simulink model "model_plane_identification_script_v1"  (R2015b)
settings: Solver=FixedStepDiscrete  StartTime=0.0  StopTime=20  RelTol=1e-3
values from neighbouring files (symbols this model uses):
  Aa = Amp_list(ii)    [amplitude_influence.m]    (also in datas.m = 1; model_validation.m = Amp_aileron2)
  Ae = Amp_list(ii)    [amplitude_influence.m]    (also in datas.m = 1; model_validation.m = Amp_elevator2)
  Ar = Amp_list(ii)    [amplitude_influence.m]    (also in datas.m = 1; model_validation.m = Amp_rudder2)
  b = 59.74    [datas.m]
  cbar = 8.32    [datas.m]
  K_wind = [0 0 0 0 0 0]'    [datas.m]
  m = 288772    [datas.m]
  Offset_Accelerometer = 57*10^-6    (= 5.7e-05)    [datas.m]
  Offset_gyro = 0.15/180*pi    (= 0.00261799387799)    [datas.m]
  Offset_velocity_angles = 0.1/180*pi    (= 0.00174532925199)    [datas.m]
  S = 510.95    [datas.m]
  Ta = 6    [datas.m]
  Te = 4    [datas.m]
  test_aileron = 1    [datas.m]    (also in model_validation.m = aileron2)
  test_elevator = 4    [datas.m]    (also in model_validation.m = elevator2)
  test_rudder = 1    [datas.m]    (also in model_validation.m = rudder2)
  Tr = 2    [datas.m]
undefined symbols (not defined in the file or in its folder): airlib, B747, DiscIntNeverNeededParam, DT, sigbuilder_block
undefined symbols (not defined in the file): Cd_0_true, Cd_alpha_true, Cd_deltae_true, Cd_q_true, Cdih_true, Cl_0_true, CL_0_true, CL_alpha_true, Cl_b_true, Cl_deltaa_true, CL_deltae_true, Cl_deltar_true, Cl_p_true, CL_q_true, Cl_r_true, CLih_true, Cm_0_true, Cm_alpha_true, Cm_deltae_true, Cm_ih_true, Cm_q_true, Cn_0_true, Cn_b_true, Cn_deltaa_true, Cn_deltar_true, Cn_p_true, Cn_r_true, Cy_0_true, Cy_b_true, Cy_deltaa_true, Cy_deltar_true, Cy_p_true, Cy_r_true, Ix, Iy, Iz, Jxy, Jxz, Jyz, V
libraries: simulink x4
(part 1 of 2)
settings Model: Creator=LiMing  LastModifiedBy=c.mathis
settings DataIOCC: LimitDataPoints=off  SaveFormat=Array  SignalLoggingSaveFormat=ModelDataLogs  SaveOutput=off  SaveTime=off
settings OptimizationCC: BlockReduction=off  BooleanDataType=off  ExpressionDepthLimit=2147483647  InitFltsAndDblsToZero=on
settings DebuggingCC: SaveWithParameterizedLinksMsg=none  UnderspecifiedInitializationDetection=Classic  MergeDetectMultiDrivingBlocksExec=none  SignalResolutionControl=TryResolveAllWithWarning  MultiTaskDSMMsg=warning  MultiTaskCondExecSysMsg=none  FcnCallInpInsideContextMsg=UseLocalSettings  StateNameClashWarn=warning
settings HardwareCC: ProdBitPerPointer=32  ProdLargestAtomicFloat=None  ProdIntDivRoundTo=Undefined  ProdEndianess=Unspecified  ProdWordSize=32  ProdHWDeviceType=32-bit Generic  TargetUnknown=on
settings GRTTargetCC: GeneratePreprocessorConditionals=Disable all  CombineOutputUpdateFcns=off  GRTInterface=on
settings ConfigComp: CovModelRefEnable=Off

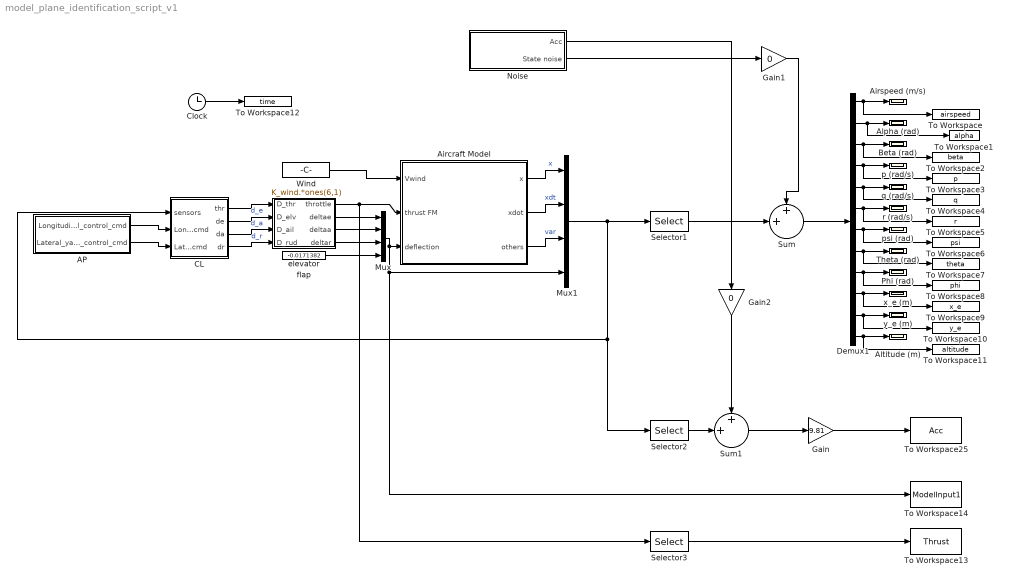
== system model_plane_identification_script_v1 ==
  AP : Subsystem
  Aircraft Model : Subsystem  AncestorBlock=airlib/DT-B747  mask(Discrete Time General Nonlinear Aircraft Model){GM1=[cbar   b   S   Ix  Iy   Iz   Jxy   Jxz  Jyz   m  0.02], CD_wind=[Cd_0_true  Cd_alpha_true  Cd_q_true  Cd_deltae_true  Cdih_true], CL_wind=[CL_0_true  CL_alpha_true  CL_q_true  CL_deltae_true  CLih_true], Cm_body=[Cm_0_true  Cm_alpha_true   Cm_q_true  Cm_deltae_true  Cm_ih_true ], CY_body=[Cy_0_true   Cy_b_true    Cy_p_true     Cy_r_true     Cy_deltaa_true    Cy_deltar_true], Cl_body=[Cl_0_true    Cl_b_true    Cl_p_true   Cl_r_true   Cl_deltaa_true   Cl_deltar_true], Cn_body=[Cn_0_true    Cn_b_true   Cn_p_true    Cn_r_true     Cn_deltaa_true   Cn_deltar_true], x0=[V  0.0464959 0   0 0 0   0 0.0464959 0   0 0 61]}
      mask prompts: GM1 "Geometry, Mass, T : [cbar   b    S    Ix   Iy   Iz   Jxy  Jxz  Jyz  m  T]"; CD_wind "Aerodynamic D-Force Derivatives : [CD0 CDa CDq CDde CDih]"; CL_wind "Aerodynamic L-Force Derivatives : [CL0 CLa CLq CLde CLih]"; Cm_body "Aerodynamic Y-Moment Derivatives : [Cm0 Cma Cmq Cmde Cmih]"; CY_body "Aerodynamic Y-Force Derivatives : [CY0 CYb CYp CYr CYda CYdr]"; Cl_body "Aerodynamic X-moment Derivatives : [Cl0 Clb Clp Clr Clda Cldr]"; Cn_body "Aerodynamic Z-moment Derivatives : [Cn0 Cnb Cnp Cnr Cnda Cndr]"; x0 "Initial Condition x0 [v alpha beta p q r psi theta phi xe ye H]"
      mask help:
      | The first input contains the wind velocity and acceleration.
      |   The second input contains external forces and moments in body axis.
      |   The third input contains the deflections of elevators, ailerons, rudder,
      |   and flaps. For a list of outputs look under the mask.
      |   NB : The International measurement system (MKS) is adopted.
      mask init:
      | AM=zeros(6,19);
      | AM(1,[1 2 9 11 12])=reshape(CD_wind,1,5);
      | AM(3,[1 2 9 11 12])=reshape(CL_wind,1,5);
      | AM(5,[1 2 9 11 12])=reshape(Cm_body,1,5);
      | AM(2,[1 5 8 10 13 14])=reshape(CY_body,1,6);
      | AM(4,[1 5 8 10 13 14])=reshape(Cl_body,1,6);
      | AM(6,[1 5 8 10 13 14])=reshape(Cn_body,1,6);
      | 
      | Ix=GM1(4);Iy=GM1(5);Iz=GM1(6);
      | Jxy=GM1(7);Jxz=GM1(8);Jyz=GM1(9);
      | 
      | detI = Ix*Iy*Iz - 2*Jxy*Jxz*Jyz - Ix*Jyz^2 - Iy*Jxz^2 - Iz*Jxy^2;
      | I1   = Iy*Iz - Jyz^2;I2   = Jxy*Iz + Jyz*Jxz;
      | I3   = Jxy*Jyz + Iy*Jxz;I4   = Ix*Iz - Jxz^2;
      | I5   = Ix*Jyz + Jxy*Jxz;I6   = Ix*Iy - Jxy^2;
      | 
      | Pl  = I1/detI; Pm = I2/detI; Pn = I3/detI;
      | Ppp = -(Jxz*I2 - Jxy*I3)/detI;Ppq = (Jxz*I1 - Jyz*I2 - (Iy-Ix)*I3)/detI;
      | Ppr = -(Jxy*I1 + (Ix-Iz)*I2 - Jyz*I3)/detI;Pqq = (Jyz*I1 - Jxy*I3)/detI;
      | Pqr = -((Iz-Iy)*I1 - Jxy*I2 + Jxz*I3)/detI;Prr = -(Jyz*I1 - Jxz*I2)/detI;
      | 
      | Ql  = I2/detI; Qm = I4/detI; Qn = I5/detI;
      | Qpp = -(Jxz*I4 - Jxy*I5)/detI;Qpq = (Jxz*I2 - Jyz*I4 - (Iy-Ix)*I5)/detI;
      | Qpr = -(Jxy*I2 + (Ix-Iz)*I4 - Jyz*I5)/detI;Qqq = (Jyz*I2 - Jxy*I5)/detI;
      | Qqr = -((Iz-Iy)*I2 - Jxy*I4 + Jxz*I5)/detI;Qrr = -(Jyz*I2 - Jxz*I4)/detI;
      | 
      | Rl  = I3/detI; Rm = I5/detI; Rn = I6/detI;
      | Rpp = -(Jxz*I5 - Jxy*I6)/detI;
      | Rpq = (Jxz*I3 - Jyz*I5 - (Iy-Ix)*I6)/detI;
      | Rpr = -(Jxy*I3 + (Ix-Iz)*I5 - Jyz*I6)/detI;
      | Rqq = (Jyz*I3 - Jxy*I6)/detI;
      | Rqr = -((Iz-Iy)*I3 - Jxy*I5 + Jxz*I6)/detI;
      | Rrr = -(Jyz*I3 - Jxz*I5)/detI;
      | 
      | GM2 = [  Pl   Pm   Pn   Ppp  Ppq  Ppr  Pqq  Pqr  Prr ;
      |                Ql  Qm   Qn   Qpp  Qpq  Qpr  Qqq  Qqr  Qrr ;
      |                Rl  Rm   Rn   Rpp  Rpq  Rpr  Rqq  Rqr  Rrr ];
      | 
      | xfix=1;
      | T=GM1(11);
      mask Help:
      | <p>
      | This block is a general nonlinear 6DOF aircraft model, with a very accurate built-in atmosphere model and constant aerodynamic derivatives.
      | The architecture of the block is largely based on the Aircraft block provided by the <A
      | HREF="http://www.mathworks.com/matlabcentral/fileexchange/loadFile.do?objectId=252&objectType=file">FDC toolbox</A> (Marc Rauw, 1993-2000).
      | </p>
      | <p>
      | The geometric and inertal data of the aircraft are entered as parameters in the first row of the mask, sampling time is the last parameter. The other six rows contains the non-dimensional aerodynamic derivatives. The last row is the initial state.
      | </p>
      | <p>
      | The first input contains the wind velocity and acceleration.
      | The second input contains external forces and moments in the aircraft body axis.
      | The third input contains the deflections of elevators, ailerons, rudder,
      | and flaps or stabilators. For a list of outputs look under the mask.
      | </p>
      | <p>
      | The control surface sign conventions are the same adopted in books such as Stevens-Lewis and Etkin, and in many flight simulators,
      | including the FDC toolbox. <br>
      | Specifically, positive elevator deflection causes negative pitching moment (Cmde &#60 0), positive rudder deflection causes negative yawing
      | moment (Cndr &#60 0), and positive aileron deflection causes negative rolling moment (Clda &#60 0). Another way to say the same thing is
      | that, the positive elevators deflection is Trailing Edge Down (TED), the positive rudder(s) deflection is Trailing Edge Left (TEL), and,
      | taking as TED the positive ailerons deflection, da=K*(da_right-da_left), with K usually equal to 1 (FDC) or 1/2.
      | </p>
      | <p>
      | Since this block is largely based on the FDC toolbox, i redirect you to the FDC Toolbox manual, for a good explanation of the underlying
      | components. Besides the mask and the fact that the aerodynamic derivatives are expressed in the stability axis, the only relevant difference
      | with the FDC toolbox is that in the computation of the aerodynamic forces, q is normalized as q*cbar/2V instead of q*cbar/V. The majority
      | of aeronautics books that i've seen use q*cbar/2V.
      | </p>
      | <p>
      | Please note that the International Measurement System is adopted. So, lengths are in meters, masses in Kg, and inertia moments in Kg*m^2.
      | Moreover, forces are in N, moments in N*m, accelerations in g, and angles in radians. For those that use the english system, here are some useful
      | conversion factors: <br>
      | 1 ft   = 0.3048 m, 1 lb   = 0.4536 Kg, 1 slug = 14.593903 Kg ,  1 slug*ft^2 = 1.355818 Kg*m^2
      | <br>
      | </p>
      | <p>
      | Finally, there is an <A HREF="http://www.aae.uiuc.edu/m-selig/apasim/Aircraft-uiuc.html">excellent source</A> of aircraft aerodynamic data
      | which is mantained by Michael S. Selig, Rob Deters, and Glen Dimock at the university of Urbana-Champaign. To use any of the given models
      | you just need to type the supplied aircraft data in the block mask.
      | </p>
      | <p>
      | <p>
      | December 2002, Giampiero Campa
      | </p>
      | </p>
      mask Display:
      | image(imread('ATR72.jpg'))
      | %disp('Discrete\nTime\nGeneral\nAircraft\nModel')
  Airspeed (m/s) : Scope
  Alpha (rad) : Scope
  Altitude (m) : Scope
  Beta (rad) : Scope
  CL : Subsystem
  Clock : Clock
      settings: Decimation=20
  Demux1 : Demux  Outputs=12
  Gain : Gain  Gain=9.81
  Gain1 : Gain  Gain=0
  Gain2 : Gain  Gain=0
  Mux : Mux
  Mux1 : Mux  Inputs=[12 12 9 4]
  Noise : Subsystem
  Phi (rad) : Scope
  Selector1 : Selector  InputPortWidth=37  IndexOptions=Index vector (dialog)  Indices=1:12  OutputSizes=1
  Selector2 : Selector  InputPortWidth=37  IndexOptions=Index vector (dialog)  Indices=28:30  OutputSizes=1
  Selector3 : Selector  InputPortWidth=6  IndexOptions=Index vector (dialog)  Indices=1  OutputSizes=1
  Sum : Sum  Inputs=++|
  Sum1 : Sum  Inputs=++|
  Theta (rad) : Scope
  To Workspace : ToWorkspace  VariableName=airspeed  SampleTime=-1
  To Workspace1 : ToWorkspace  VariableName=alpha  SampleTime=-1
  To Workspace10 : ToWorkspace  VariableName=y_e  SampleTime=-1
  To Workspace11 : ToWorkspace  VariableName=altitude  SampleTime=-1
  To Workspace12 : ToWorkspace  VariableName=time  SampleTime=-1
  To Workspace13 : ToWorkspace  VariableName=Thrust  SaveFormat=Structure With Time  SampleTime=-1
  To Workspace14 : ToWorkspace  VariableName=ModelInput1  SaveFormat=Structure With Time  SampleTime=-1
  To Workspace2 : ToWorkspace  VariableName=beta  SampleTime=-1
  To Workspace25 : ToWorkspace  VariableName=Acc  SampleTime=-1
  To Workspace3 : ToWorkspace  VariableName=p  SampleTime=-1
  To Workspace4 : ToWorkspace  VariableName=q  SampleTime=-1
  To Workspace5 : ToWorkspace  VariableName=r  SampleTime=-1
  To Workspace6 : ToWorkspace  VariableName=psi  SampleTime=-1
  To Workspace7 : ToWorkspace  VariableName=theta  SampleTime=-1
  To Workspace8 : ToWorkspace  VariableName=phi  SampleTime=-1
  To Workspace9 : ToWorkspace  VariableName=x_e  SampleTime=-1
  Wind : Constant  Value=K_wind.*ones(6,1)
  elevator : Subsystem
      mask Display: disp('Engine &\nCable &\nActuator')
  flap : Constant  Value=-0.0171382
  p (rad/s) : Scope
  psi (rad) : Scope
  q (rad/s) : Scope
  r (rad/s) : Scope
  x_e (m) : Scope
  y_e (m) : Scope
  wires:
  elevator/3(deltaa) -> Mux/2
  elevator/4(deltar) -> Mux/3
  elevator/2(deltae) -> Mux/1
  CL/2(de) -> elevator/2(D_elv)  "d_e"
  CL/3(da) -> elevator/3(D_ail)  "d_a"
  CL/4(dr) -> elevator/4(D_rud)  "d_r"
  elevator/1(throttle) -> Aircraft Model/2(thrust FM), Selector3/1
  Demux1/1 -> Airspeed (m/s)/1, To Workspace/1
  Demux1/2 -> To Workspace1/1, Alpha (rad)/1
  Demux1/3 -> Beta (rad)/1, To Workspace2/1
  Demux1/5 -> q (rad/s)/1, To Workspace4/1
  Demux1/6 -> r (rad/s)/1, To Workspace5/1
  Demux1/7 -> psi (rad)/1, To Workspace6/1
  Demux1/8 -> Theta (rad)/1, To Workspace7/1
  Demux1/9 -> Phi (rad)/1, To Workspace8/1
  Demux1/10 -> x_e (m)/1, To Workspace9/1
  Demux1/11 -> y_e (m)/1, To Workspace10/1
  Demux1/12 -> Altitude (m)/1, To Workspace11/1
  CL/1(thr) -> elevator/1(D_thr)
  flap/1 -> Mux/4
  Wind/1 -> Aircraft Model/1(" Vwind")
  Aircraft Model/1(x) -> Mux1/1  "x"
  Aircraft Model/2(xdot) -> Mux1/2  "xdt"
  Aircraft Model/3(others) -> Mux1/3  "var"
  Clock/1 -> To Workspace12/1
  AP/1(Longitudinal_control_cmd) -> CL/2(Longitudinal_control_cmd)
  AP/2(Lateral_yaw_control_cmd) -> CL/3(Lateral_yaw_control_cmd)
  Selector2/1 -> Sum1/2
  Gain/1 -> To Workspace25/1
  Mux1/1 -> CL/1(sensors), Selector2/1, Selector1/1
  Sum/1 -> Demux1/1
  Selector1/1 -> Sum/2
  Sum1/1 -> Gain/1
  Mux/1 -> To Workspace14/1, Mux1/4, Aircraft Model/3(deflection)
  Selector3/1 -> To Workspace13/1
  Noise/1("Acc ") -> Gain2/1
  Demux1/4 -> p (rad/s)/1, To Workspace3/1
  Noise/2(State noise) -> Gain1/1
  Gain2/1 -> Sum1/1
  Gain1/1 -> Sum/1

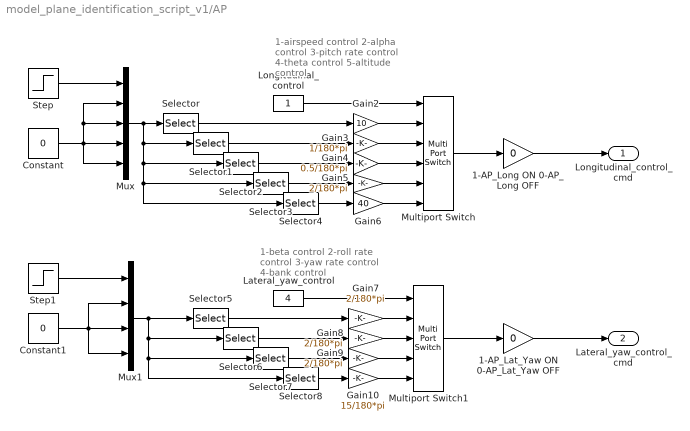
== system model_plane_identification_script_v1/AP ==
  note: 1-airspeed control
      | 2-alpha control
      | 3-pitch rate control
      | 4-theta control
      | 5-altitude control
  note: 1-beta control
      | 2-roll rate control
      | 3-yaw rate control
      | 4-bank control
  1-AP_Lat_Yaw ON 0-AP_Lat_Yaw OFF : Gain  Gain=0
  1-AP_Long ON 0-AP_Long OFF : Gain  Gain=0
  Constant : Constant  Value=0
  Constant1 : Constant  Value=0
  Gain10 : Gain  Gain=15/180*pi
  Gain2 : Gain  Gain=10
  Gain3 : Gain  Gain=1/180*pi
  Gain4 : Gain  Gain=0.5/180*pi
  Gain{5,7..9} (4 alike) : Gain  Gain=2/180*pi
  Gain6 : Gain  Gain=40
  Lateral_yaw_control : Constant  Value=4
  Longitudinal_control : Constant
  Multiport Switch : MultiPortSwitch  Inputs=5
  Multiport Switch1 : MultiPortSwitch  Inputs=4
  Mux : Mux  Inputs=5
  Mux1 : Mux
  Selector : Selector  InputPortWidth=5  IndexOptions=Index vector (dialog)  Indices=[1 2 3 4 5]  OutputSizes=1
  Selector1 : Selector  InputPortWidth=5  IndexOptions=Index vector (dialog)  Indices=[2 1 3 4 5]  OutputSizes=1
  Selector2 : Selector  InputPortWidth=5  IndexOptions=Index vector (dialog)  Indices=[3 2 1 4 5]  OutputSizes=1
  Selector3 : Selector  InputPortWidth=5  IndexOptions=Index vector (dialog)  Indices=[4 2 3 1 5]  OutputSizes=1
  Selector4 : Selector  InputPortWidth=5  IndexOptions=Index vector (dialog)  Indices=[5 2 3 4 1]  OutputSizes=1
  Selector5 : Selector  InputPortWidth=4  IndexOptions=Index vector (dialog)  Indices=[1 2 3 4]  OutputSizes=1
  Selector6 : Selector  InputPortWidth=4  IndexOptions=Index vector (dialog)  Indices=[2 1 3 4]  OutputSizes=1
  Selector7 : Selector  InputPortWidth=4  IndexOptions=Index vector (dialog)  Indices=[3 2 1 4]  OutputSizes=1
  Selector8 : Selector  InputPortWidth=4  IndexOptions=Index vector (dialog)  Indices=[4 2 3 1]  OutputSizes=1
  Step : Step  Time=20  SampleTime=0
  Step1 : Step  Time=20  SampleTime=0
  Longitudinal_control_cmd : Outport
  Lateral_yaw_control_cmd : Outport  Port=2
  wires:
  Step/1 -> Mux/1
  Constant/1 -> Mux/4, Mux/5, Mux/2, Mux/3
  Mux/1 -> Selector/1, Selector1/1, Selector2/1, Selector3/1, Selector4/1
  Selector/1 -> Gain2/1
  Longitudinal_control/1 -> Multiport Switch/1
  Selector1/1 -> Gain3/1
  Selector2/1 -> Gain4/1
  Selector3/1 -> Gain5/1
  Selector4/1 -> Gain6/1
  Multiport Switch/1 -> 1-AP_Long ON 0-AP_Long OFF/1
  Constant1/1 -> Mux1/3, Mux1/2, Mux1/4
  Mux1/1 -> Selector7/1, Selector8/1, Selector6/1, Selector5/1
  Selector5/1 -> Gain7/1
  Lateral_yaw_control/1 -> Multiport Switch1/1
  Selector6/1 -> Gain8/1
  Selector7/1 -> Gain9/1
  Selector8/1 -> Gain10/1
  Multiport Switch1/1 -> 1-AP_Lat_Yaw ON 0-AP_Lat_Yaw OFF/1
  Step1/1 -> Mux1/1
  1-AP_Long ON 0-AP_Long OFF/1 -> Longitudinal_control_cmd/1
  1-AP_Lat_Yaw ON 0-AP_Lat_Yaw OFF/1 -> Lateral_yaw_control_cmd/1
  Gain3/1 -> Multiport Switch/3
  Gain4/1 -> Multiport Switch/4
  Gain5/1 -> Multiport Switch/5
  Gain6/1 -> Multiport Switch/6
  Gain7/1 -> Multiport Switch1/2
  Gain8/1 -> Multiport Switch1/3
  Gain9/1 -> Multiport Switch1/4
  Gain10/1 -> Multiport Switch1/5
  Gain2/1 -> Multiport Switch/2

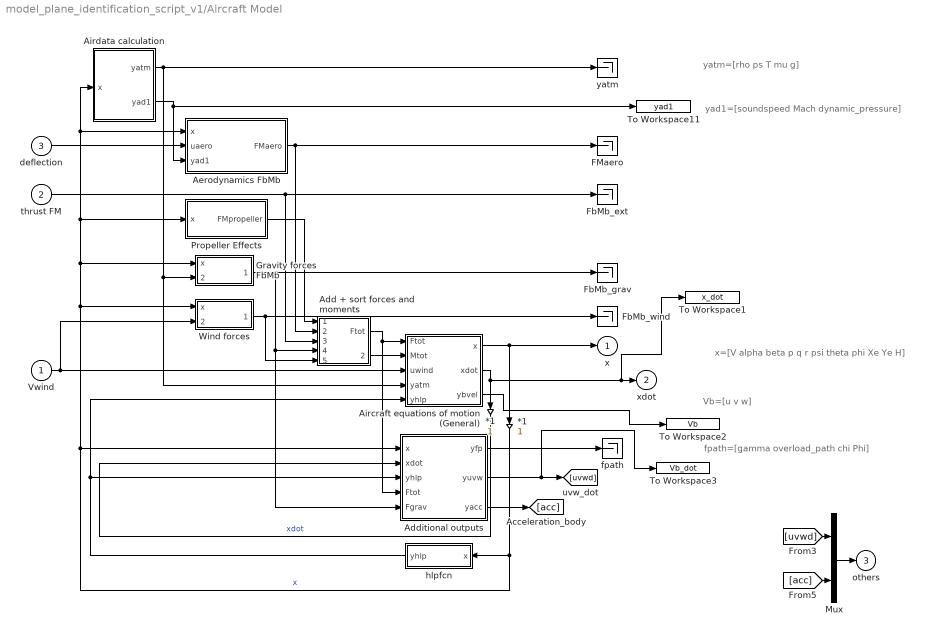
== system model_plane_identification_script_v1/Aircraft Model ==
  note: x=[V alpha beta p q r psi theta phi Xe Ye H]
  note: Vb=[u v w]
  note: fpath=[gamma overload_path chi Phi]
  note: yatm=[rho ps T mu g]
  note: yad1=[soundspeed Mach dynamic_pressure]
  " Vwind" : Inport
  thrust FM : Inport  Port=2
  deflection : Inport  Port=3
  " *1" : Gain  SaturateOnIntegerOverflow=on  OutDataTypeStr=Inherit: Same as input  ParamDataTypeStr=Inherit: Same as input
  *1 : Gain  SaturateOnIntegerOverflow=on  OutDataTypeStr=Inherit: Same as input  ParamDataTypeStr=Inherit: Same as input
  Add + sort forces and moments : Subsystem  mask(FMsort){}
      mask help: Forces and Moments sorting block
      mask Display: disp('FMsort')
  Additional outputs : Subsystem
      mask Display: disp('Additional Outputs')
  Aerodynamics FbMb : Subsystem
      mask Display: disp('Aerodynamics FbMb')
  Aircraft equations of motion (General) : Subsystem
      mask Display: disp('Eqation of Motion')
  Airdata calculation : Subsystem
      mask Display: disp('Airdata')
  FMaero : Terminator
  FbMb_ext : Terminator
  FbMb_grav : Terminator
  FbMb_wind : Terminator
  Gravity forces FbMb : Subsystem  mask(Gravity){m=GM1(10)}
      mask prompts: m "Mass of the aircraft [kg]:"
      mask help: Gravity forces.
      mask Display: disp('Gravity')
  Mux : Mux  Inputs=[3 6]
  Propeller Effects : Subsystem
      mask Display: disp('Propeller Effects')
  To Workspace1 : ToWorkspace  VariableName=x_dot  SampleTime=-1
  To Workspace11 : ToWorkspace  VariableName=yad1  SampleTime=-1
  To Workspace2 : ToWorkspace  VariableName=Vb  SampleTime=-1
  To Workspace3 : ToWorkspace  VariableName=Vb_dot  SampleTime=-1
  Wind forces : Subsystem  mask(fwind){m=GM1(10)}
      mask prompts: m "Mass of the aircraft [kg]:"
      mask help: Forces due to non-steady atmosphere.
      mask Display: disp('Fwind')
  fpath : Terminator
  hlpfcn : Subsystem  mask(Hlpfcn){}
      mask help: Help sines and cosines
      mask Display: disp('hlpfcn')
  yatm : Terminator
  x : Outport
  xdot : Outport  Port=2
  others : Outport  Port=3
  wires:
  Mux/1 -> others/1
  [acc] -> Mux/2
  [uvwd] -> Mux/1
  Additional outputs/2(yuvw) -> To Workspace3/1, [uvwd]
  Add + sort forces and moments/2(Mtot) -> Aircraft equations of motion (General)/2(Mtot)
  Aircraft equations of motion (General)/1(x) -> " *1"/1, x/1
  Aircraft equations of motion (General)/2(xdot) -> *1/1, To Workspace1/1, xdot/1
  " *1"/1 -> Gravity forces FbMb/1(x), Airdata calculation/1(x), Aerodynamics FbMb/1(x), Propeller Effects/1(x), Wind forces/1(x), Additional outputs/1(x), hlpfcn/1(x)  "x"
  Gravity forces FbMb/1(Fgrav) -> FbMb_grav/1, Additional outputs/5(Fgrav), Add + sort forces and moments/4(Fgrav)
  *1/1 -> Additional outputs/2(xdot)  "xdot"
  " Vwind"/1 -> Wind forces/2(uwind), Aircraft equations of motion (General)/3(uwind)
  hlpfcn/1(yhlp) -> Additional outputs/3(yhlp), Aircraft equations of motion (General)/5(yhlp)
  Aerodynamics FbMb/1(FMaero) -> Add + sort forces and moments/2(FMaero), FMaero/1
  Wind forces/1(Fwind) -> Add + sort forces and moments/5(Fwind), FbMb_wind/1
  Additional outputs/3(yacc) -> [acc]
  Airdata calculation/1(yatm) -> yatm/1, Gravity forces FbMb/2(yatm), Aircraft equations of motion (General)/4(yatm)
  Airdata calculation/2(yad1) -> To Workspace11/1, Aerodynamics FbMb/3(yad1)
  Additional outputs/1(yfp) -> fpath/1
  Aircraft equations of motion (General)/3(ybvel) -> To Workspace2/1
  deflection/1 -> Aerodynamics FbMb/2(uaero)
  thrust FM/1 -> FbMb_ext/1, Add + sort forces and moments/3(FMprop)
  Add + sort forces and moments/1(Ftot) -> Aircraft equations of motion (General)/1(Ftot), Additional outputs/4(Ftot)
  Propeller Effects/1(FMpropeller) -> Add + sort forces and moments/1(FM_propeller)

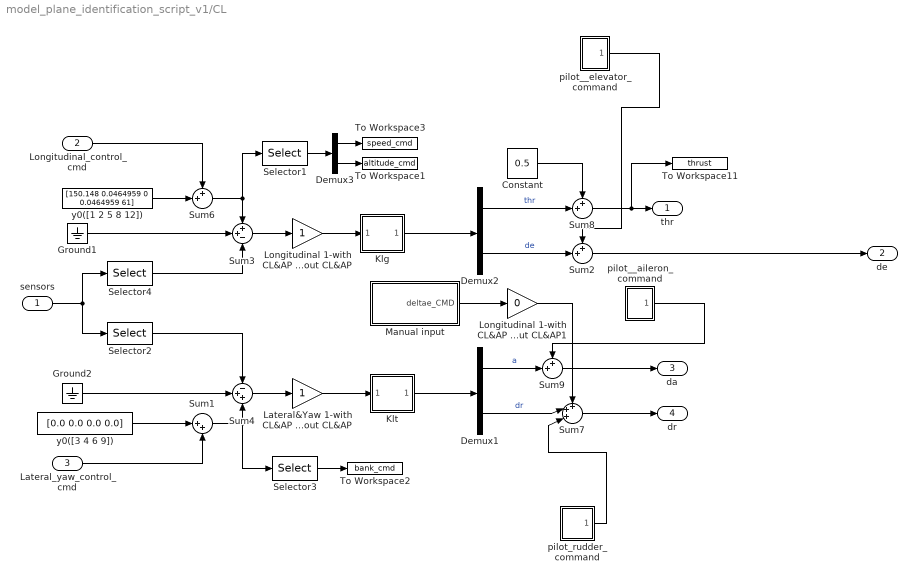
== system model_plane_identification_script_v1/CL ==
  sensors : Inport
  Longitudinal_control_cmd : Inport  Port=2
  Lateral_yaw_control_cmd : Inport  Port=3
  Constant : Constant  Value=0.5
  Demux1 : Demux  Outputs=2
  Demux2 : Demux  Outputs=2
  Demux3 : Demux  Outputs=2
  Ground1 : Ground
  Ground2 : Ground
  "Klg " : Subsystem  mask(State Space){M=[0.1942   -0.8227    0.0057    0.6253    0.0090;  0.0283    7.9374   -5.0871  -16.2986   -0.0437]}
      mask prompts: M "Matrix"
      mask Display: disp('Matrix\nGain')
  "Klt " : Subsystem  mask(State Space){M=[0.2844   -0.1878   -0.2314   -0.1641; 1.1821   -0.4567   -1.8328   -0.4900]}
      mask prompts: M "Matrix"
      mask Display: disp('Matrix\nGain')
  Lateral&Yaw 1-with CL&AP 0-without CL&AP : Gain
  Longitudinal 1-with CL&AP 0-without CL&AP : Gain
  Longitudinal 1-with CL&AP 0-without CL&AP1 : Gain  Gain=0
  Manual input : Subsystem  Tag=STV Subsys  LoadFcn=sigbuilder_block('load');  StartFcn=sigbuilder_block('start');  StopFcn=sigbuilder_block('stop');  ClipboardFcn=sigbuilder_block('clipboard');  mask(Sigbuilder block){}
      mask help: Simulink:masks:SigbuilderBlock_MD
      mask init:
      | if ~strcmp(get_param(bdroot(gcbh),'SimulationStatus'),'stopped') tuvar = sigbuilder_block('maskInit'); end
      settings: CopyFcn=sigbuilder_block('copy');  DeleteFcn=sigbuilder_block('delete');  ModelCloseFcn=sigbuilder_block('modelClose');  PreSaveFcn=sigbuilder_block('preSave');  PauseFcn=sigbuilder_block('pause');  ContinueFcn=sigbuilder_block('continue');  NameChangeFcn=sigbuilder_block('namechange');  OpenFcn=sigbuilder_block('open',[301.5 193.5 843.75 381.75 ]);  CloseFcn=sigbuilder_block('close');
      mask Display: plot(0, 0, 100, 100,[2, 2, 32, 32, 2], [68, 8, 8, 68, 68],[32, 2], [38, 38], [32, 19, 2],[53, 60, 44], [32, 17, 17, 2],[16, 16, 31, 31]);txt = getActiveGroup(gcbh);text(2, 100, txt,'verticalAlignment', 'top');
  Selector1 : Selector  InputPortWidth=5  IndexOptions=Index vector (dialog)  Indices=[1 5]  OutputSizes=1
  Selector2 : Selector  InputPortWidth=37  IndexOptions=Index vector (dialog)  Indices=[3 4 6 9]  OutputSizes=1
  Selector3 : Selector  InputPortWidth=4  IndexOptions=Index vector (dialog)  Indices=[4]  OutputSizes=1
  Selector4 : Selector  InputPortWidth=37  IndexOptions=Index vector (dialog)  Indices=[1 2 5 8 12]  OutputSizes=1
  Sum1 : Sum  Inputs=|++  SaturateOnIntegerOverflow=on  InputSameDT=on  OutDataTypeStr=Inherit: Same as first input
  Sum{2,6,8..9} (4 alike) : Sum  Inputs=++|  SaturateOnIntegerOverflow=on  InputSameDT=on  OutDataTypeStr=Inherit: Same as first input
  Sum3 : Sum  Inputs=++-  SaturateOnIntegerOverflow=on  InputSameDT=on  OutDataTypeStr=Inherit: Same as first input
  Sum4 : Sum  Inputs=-++  SaturateOnIntegerOverflow=on  InputSameDT=on  OutDataTypeStr=Inherit: Same as first input
  Sum7 : Sum  Inputs=+++|  SaturateOnIntegerOverflow=on  InputSameDT=on  OutDataTypeStr=Inherit: Same as first input
  To Workspace1 : ToWorkspace  VariableName=altitude_cmd  SampleTime=-1
  To Workspace11 : ToWorkspace  VariableName=thrust  SampleTime=-1
  To Workspace2 : ToWorkspace  VariableName=bank_cmd  SampleTime=-1
  To Workspace3 : ToWorkspace  VariableName=speed_cmd  SampleTime=-1
  pilot__aileron_command : Subsystem
  pilot__elevator_command : Subsystem
  pilot_rudder_command : Subsystem
  y0([1 2 5 8 12]) : Constant  Value="[150.148  0.0464959 0 0.0464959 61]"
  y0([3 4 6 9]) : Constant  Value=[0.0 0.0 0.0 0.0]
  thr : Outport
  de : Outport  Port=2
  da : Outport  Port=3
  dr : Outport  Port=4
  wires:
  sensors/1 -> Selector4/1, Selector2/1
  Selector4/1 -> Sum3/3
  Sum3/1 -> Longitudinal 1-with CL&AP 0-without CL&AP/1
  Ground1/1 -> Sum3/2
  "Klg "/1(Out1) -> Demux2/1
  Sum4/1 -> Lateral&Yaw 1-with CL&AP 0-without CL&AP/1
  Ground2/1 -> Sum4/2
  Selector2/1 -> Sum4/1
  Lateral_yaw_control_cmd/1 -> Sum1/2
  y0([3 4 6 9])/1 -> Sum1/1
  Sum1/1 -> Sum4/3, Selector3/1
  Longitudinal_control_cmd/1 -> Sum6/1
  y0([1 2 5 8 12])/1 -> Sum6/2
  Sum6/1 -> Sum3/1, Selector1/1
  Longitudinal 1-with CL&AP 0-without CL&AP/1 -> "Klg "/1(In1)
  Manual input/1(deltae_CMD) -> Longitudinal 1-with CL&AP 0-without CL&AP1/1
  Selector1/1 -> Demux3/1
  Demux3/2 -> To Workspace1/1
  Demux3/1 -> To Workspace3/1
  Selector3/1 -> To Workspace2/1
  Demux2/1 -> Sum8/2  "thr"
  Constant/1 -> Sum8/1
  Sum8/1 -> To Workspace11/1, thr/1
  Demux2/2 -> Sum2/2  "de"
  Sum2/1 -> de/1
  pilot__elevator_command/1(Out1) -> Sum2/1
  "Klt "/1(Out1) -> Demux1/1
  Lateral&Yaw 1-with CL&AP 0-without CL&AP/1 -> "Klt "/1(In1)
  Longitudinal 1-with CL&AP 0-without CL&AP1/1 -> Sum7/1
  Demux1/2 -> Sum7/2  "dr"
  Sum7/1 -> dr/1
  pilot_rudder_command/1(Out1) -> Sum7/3
  Demux1/1 -> Sum9/2  "a"
  Sum9/1 -> da/1
  pilot__aileron_command/1(Out1) -> Sum9/1

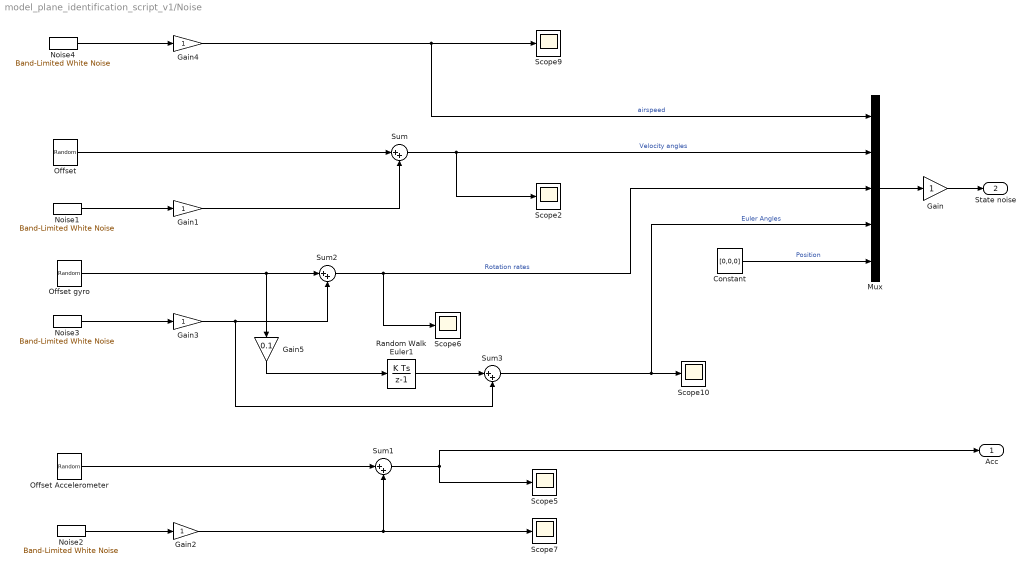
== system model_plane_identification_script_v1/Noise ==
  Constant : Constant  Value=[0,0,0]
  Gain{,1..4} (5 alike) : Gain
  Gain5 : Gain  Gain=0.1
  Mux : Mux  Inputs=5
  Noise1 : simulink/Sources/Band-Limited White Noise  Cov=Noise_power_velocity_angles  Ts=0.02  seed=1:2
  Noise2 : simulink/Sources/Band-Limited White Noise  Cov=Noise_power_Accelerometer  Ts=0.02  seed=2
  Noise3 : simulink/Sources/Band-Limited White Noise  Cov=Noise_power_gyro  Ts=0.02  seed=2
  Noise4 : simulink/Sources/Band-Limited White Noise  Cov=Noise_power_airspeed  Ts=0.02  seed=1
  Offset : UniformRandomNumber  Minimum=-Offset_velocity_angles  Maximum=Offset_velocity_angles  Seed=1:2  SampleTime=0.02
  Offset Accelerometer : UniformRandomNumber  Minimum=-Offset_Accelerometer  Maximum=Offset_Accelerometer  Seed=1:3  SampleTime=0.02
  Offset gyro : UniformRandomNumber  Minimum=-Offset_gyro  Maximum=Offset_gyro  Seed=1:3  SampleTime=0.02
  Random Walk Euler1 : DiscreteIntegrator  gainval=1  InitialConditionSetting=State (most efficient)  SampleTime=-1  ICPrevOutput=DiscIntNeverNeededParam  ICPrevScaledInput=DiscIntNeverNeededParam
  Scope{2,5..7,9..10} (6 alike) : Scope
  Sum{,1..3} (4 alike) : Sum  Inputs=|++
  "Acc " : Outport
  State noise : Outport  Port=2
  wires:
  Noise1/1 -> Gain1/1
  Offset/1 -> Sum/1
  Sum/1 -> Mux/2, Scope2/1  "Velocity angles"
  Noise2/1 -> Gain2/1
  Gain2/1 -> Scope7/1, Sum1/2
  Offset Accelerometer/1 -> Sum1/1
  Noise3/1 -> Gain3/1
  Gain3/1 -> Sum3/2, Sum2/2
  Offset gyro/1 -> Sum2/1, Gain5/1
  Sum2/1 -> Scope6/1, Mux/3  "Rotation rates"
  Sum1/1 -> Scope5/1, "Acc "/1
  Noise4/1 -> Gain4/1
  Gain4/1 -> Mux/1, Scope9/1  "airspeed"
  Constant/1 -> Mux/5  "Position"
  Mux/1 -> Gain/1
  Sum3/1 -> Scope10/1, Mux/4  "Euler Angles"
  Gain1/1 -> Sum/2
  Gain5/1 -> Random Walk Euler1/1
  Random Walk Euler1/1 -> Sum3/1
  Gain/1 -> State noise/1

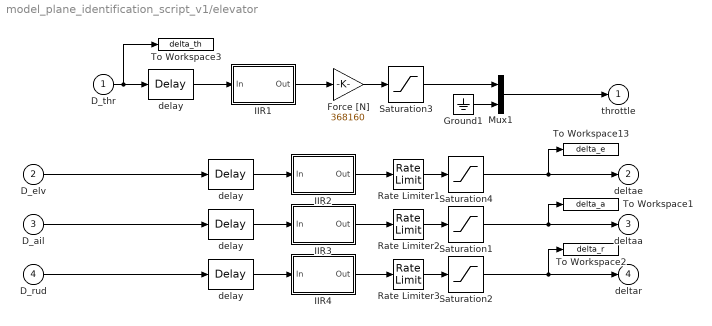
== system model_plane_identification_script_v1/elevator ==
  D_thr : Inport
  D_elv : Inport  Port=2
  D_ail : Inport  Port=3
  D_rud : Inport  Port=4
  " delay" : TransportDelay  DelayTime=0.03  InitialOutput=-1.71374e-004
  " delay " : TransportDelay  DelayTime=0.03  InitialOutput=0.490154
  Force [N] : Gain  Gain=368160  SaturateOnIntegerOverflow=on  OutDataTypeStr=Inherit: Same as input  ParamDataTypeStr=Inherit: Same as input
  Ground1 : Ground
  IIR1 : Subsystem  mask(Discrete Time First Order IIR){ni=1, a=4, x0=0.490154, T=0.02}
      mask prompts: ni "Number of Channels"; a "Cutoff Frequency (a)"; x0 "Initial Condition"; T "Sample Time"
      mask help:
      | Each channel has the transfer function
      |   (1-exp(-aT))/(1-exp(-aT)(z^-1)) which is a good
      |   (pz-matched) approximation of a/(s+a) if 10*a*T<pi
      mask init:
      | A=[];B=[];C=[];D=[];
      | for i=1:ni,
      | A=[A,zeros(size(A,1),1);zeros(1,size(A,2)),exp(-a*T)];
      | B=[B,zeros(size(B,1),1);zeros(1,size(B,2)),1-exp(-a*T)];
      | C=[C,zeros(size(C,1),1);zeros(1,size(C,2)),exp(-a*T)];
      | D=[D,zeros(size(D,1),1);zeros(1,size(D,2)),1-exp(-a*T)];
      | end
      mask Help:
      | <p>
      |   Each channel has the transfer function
      |   (1-exp(-aT))/(1-exp(-aT)(z^-1)) which is a good
      |   (pz-matched) approximation of a/(s+a) if 10*a*T<pi
      | </p>
      mask Display: dpoly(a,[1 a],'s')
  IIR2 : Subsystem  mask(Discrete Time First Order IIR){ni=1, a=15, x0=-1.71374e-004, T=0.02}
      mask prompts: ni "Number of Channels"; a "Cutoff Frequency (a)"; x0 "Initial Condition"; T "Sample Time"
      mask help:
      | Each channel has the transfer function
      |   (1-exp(-aT))/(1-exp(-aT)(z^-1)) which is a good
      |   (pz-matched) approximation of a/(s+a) if 10*a*T<pi
      mask init: same as model_plane_identification_script_v1/elevator/IIR1
      mask Help:
      | <p>
      |   Each channel has the transfer function
      |   (1-exp(-aT))/(1-exp(-aT)(z^-1)) which is a good
      |   (pz-matched) approximation of a/(s+a) if 10*a*T<pi
      | </p>
      mask Display: dpoly(a,[1 a],'s')
  IIR3 : Subsystem  mask(Discrete Time First Order IIR){ni=1, a=15, x0=0, T=0.02}
      mask prompts: ni "Number of Channels"; a "Cutoff Frequency (a)"; x0 "Initial Condition"; T "Sample Time"
      mask help:
      | Each channel has the transfer function
      |   (1-exp(-aT))/(1-exp(-aT)(z^-1)) which is a good
      |   (pz-matched) approximation of a/(s+a) if 10*a*T<pi
      mask init: same as model_plane_identification_script_v1/elevator/IIR1
      mask Help:
      | <p>
      |   Each channel has the transfer function
      |   (1-exp(-aT))/(1-exp(-aT)(z^-1)) which is a good
      |   (pz-matched) approximation of a/(s+a) if 10*a*T<pi
      | </p>
      mask Display: dpoly(a,[1 a],'s')
  IIR4 : Subsystem  mask(Discrete Time First Order IIR){ni=1, a=15, x0=0, T=0.02}
      mask prompts: ni "Number of Channels"; a "Cutoff Frequency (a)"; x0 "Initial Condition"; T "Sample Time"
      mask help:
      | Each channel has the transfer function
      |   (1-exp(-aT))/(1-exp(-aT)(z^-1)) which is a good
      |   (pz-matched) approximation of a/(s+a) if 10*a*T<pi
      mask init: same as model_plane_identification_script_v1/elevator/IIR1
      mask Help:
      | <p>
      |   Each channel has the transfer function
      |   (1-exp(-aT))/(1-exp(-aT)(z^-1)) which is a good
      |   (pz-matched) approximation of a/(s+a) if 10*a*T<pi
      | </p>
      mask Display: dpoly(a,[1 a],'s')
  Mux1 : Mux  Inputs=[1 5]
  Rate Limiter1 : RateLimiter  RisingSlewLimit=100*pi/180  FallingSlewLimit=-100*pi/180
  Rate Limiter2 : RateLimiter  RisingSlewLimit=100*pi/180  FallingSlewLimit=-100*pi/180
  Rate Limiter3 : RateLimiter  RisingSlewLimit=100*pi/180  FallingSlewLimit=-100*pi/180
  Saturation1 : Saturate  UpperLimit=20*pi/180  LowerLimit=-20*pi/180
  Saturation2 : Saturate  UpperLimit=20*pi/180  LowerLimit=-20*pi/180
  Saturation3 : Saturate  UpperLimit=245440  LowerLimit=0
  Saturation4 : Saturate  UpperLimit=20*pi/180  LowerLimit=-20*pi/180
  To Workspace1 : ToWorkspace  VariableName=delta_a  SampleTime=-1
  To Workspace13 : ToWorkspace  VariableName=delta_e  SampleTime=-1
  To Workspace2 : ToWorkspace  VariableName=delta_r  SampleTime=-1
  To Workspace3 : ToWorkspace  VariableName=delta_th  SampleTime=-1
  delay : TransportDelay  DelayTime=0.03
  "delay " : TransportDelay  DelayTime=0.03
  throttle : Outport
  deltae : Outport  Port=2
  deltaa : Outport  Port=3
  deltar : Outport  Port=4
  wires:
  IIR2/1(Out) -> Rate Limiter1/1
  Saturation4/1 -> deltae/1, To Workspace13/1
  IIR3/1(Out) -> Rate Limiter2/1
  Saturation1/1 -> deltaa/1, To Workspace1/1
  IIR4/1(Out) -> Rate Limiter3/1
  Saturation2/1 -> deltar/1, To Workspace2/1
  Rate Limiter1/1 -> Saturation4/1
  Rate Limiter2/1 -> Saturation1/1
  Rate Limiter3/1 -> Saturation2/1
  Saturation3/1 -> Mux1/1
  Ground1/1 -> Mux1/2
  D_thr/1 -> " delay "/1, To Workspace3/1
  IIR1/1(Out) -> Force [N]/1
  Force [N]/1 -> Saturation3/1
  " delay "/1 -> IIR1/1(In)
  " delay"/1 -> IIR2/1(In)
  delay/1 -> IIR3/1(In)
  "delay "/1 -> IIR4/1(In)
  D_elv/1 -> " delay"/1
  D_ail/1 -> delay/1
  D_rud/1 -> "delay "/1
  Mux1/1 -> throttle/1

== system model_plane_identification_script_v1/Aircraft Model/Add + sort forces and moments ==
  FM_propeller : Inport
  FMaero : Inport  Port=2
  FMprop : Inport  Port=3
  Fgrav : Inport  Port=4
  Fwind : Inport  Port=5
  Demux : Demux  Outputs=[3 3]
  Demux1 : Demux  Outputs=[3 3]
  Demux2 : Demux  Outputs=[3 3]
  Sum1 : Sum  Inputs=+++  SaturateOnIntegerOverflow=on  InputSameDT=on  OutDataTypeStr=Inherit: Same as first input
  Sum3 : Sum  Inputs=+++++  SaturateOnIntegerOverflow=on  InputSameDT=on  OutDataTypeStr=Inherit: Same as first input
  Ftot : Outport
  Mtot : Outport  Port=2
  wires:
  Fwind/1 -> Sum3/4
  Demux/1 -> Sum3/1
  Sum1/1 -> Mtot/1
  Sum3/1 -> Ftot/1
  Demux1/1 -> Sum3/2
  Fgrav/1 -> Sum3/3
  Demux/2 -> Sum1/1
  Demux1/2 -> Sum1/2
  FMprop/1 -> Demux1/1
  FMaero/1 -> Demux/1
  FM_propeller/1 -> Demux2/1
  Demux2/1 -> Sum3/5
  Demux2/2 -> Sum1/3

== system model_plane_identification_script_v1/Aircraft Model/Additional outputs ==
  note: Body-axes accelerations
      | and specific forces
  note: du/dt, dv/dt, dw/dt
      | (output equations!)
  note: Flightpath
      | variables
  x : Inport
  xdot : Inport  Port=2
  yhlp : Inport  Port=3
  Ftot : Inport  Port=4
  Fgrav : Inport  Port=5
  accel : Subsystem  mask(accel){m=GM1(10)}
      mask prompts: m "Mass of the aircraft [kg]:"
      mask help:
      | Body axes accelerations and
      | specific forces.
      mask Display: disp('Accel')
  fp : Subsystem  mask(Flpath){alpha0=x0(2)}
      mask prompts: alpha0 "Initial value of angle of attack, alpha0:"
      mask help: Flightpath related parameters.
      mask Display: disp('flpath')
  uvwdot : Subsystem  mask(uvwdot){}
      mask help: Calculation of du/dt, dv/dt, and dw/dt.
      mask Display: disp('uvwdot')
  yfp : Outport
  yuvw : Outport  Port=2
  yacc : Outport  Port=3
  wires:
  Fgrav/1 -> accel/2(Fgrav)
  x/1 -> uvwdot/1(x), fp/1(x)
  xdot/1 -> uvwdot/2(xdot), fp/2(xdot)
  accel/1(yacc) -> yacc/1
  Ftot/1 -> accel/1(Ftot)
  yhlp/1 -> uvwdot/3(yhlp)
  uvwdot/1(yuvw = [udot; vdot; wdot]) -> yuvw/1
  fp/1(yfp) -> yfp/1

== system model_plane_identification_script_v1/Aircraft Model/Aerodynamics FbMb ==
  x : Inport
  uaero : Inport  Port=2
  yad1 : Inport  Port=3
  Caero : Terminator
  aero : Subsystem  mask(Aeromod){}
      mask help: Aerodynamic model of the DHC-2 'Beaver'.
      mask Display: disp('Aeromod\n(General)')
  dl : Subsystem  mask(Dimless){cbar=GM1(1), b=GM1(2)}
      mask prompts: cbar "Mean aerodynamic chord [m]:"; b "Wing span [m]:"
      mask help: Dimensionless rotational velocities.
      mask Display: disp('Dimless')
  fmdims : Subsystem  mask(FMdims){cbar=GM1(1), b=GM1(2), S=GM1(3)}
      mask prompts: cbar "Mean aerodynamic chord [m]:"; b "Wing span [m]:"; S "Wing surface [m^2]:"
      mask help:
      | Calculate forces and moments from
      | dimensionless derivatives.
      mask Display: disp('FMdims')
  ydl : Terminator
  FMaero : Outport
  wires:
  fmdims/1(Forces and moments) -> FMaero/1
  yad1/1 -> fmdims/1(yad1)
  uaero/1 -> aero/2(uaero)
  x/1 -> aero/1(x), dl/1(x)
  dl/1(ydl) -> aero/3(ydl), ydl/1
  aero/1(Caero) -> fmdims/2(Force / moment derivatives), Caero/1

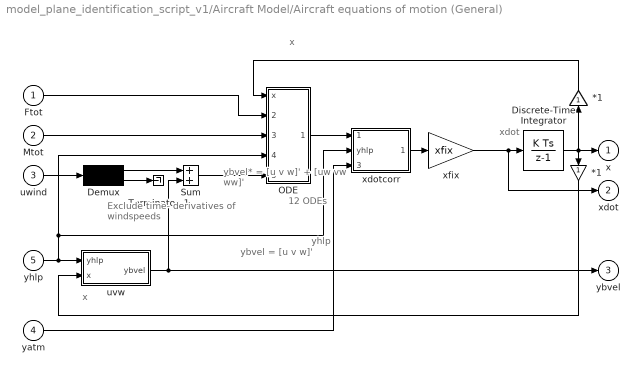
== system model_plane_identification_script_v1/Aircraft Model/Aircraft equations of motion (General) ==
  note: 12 ODEs
  note: ybvel = [u v w]'
  note: yhlp
  note: x
  note: x
  note: xdot
  note: ybvel* =
      | [u v w]' +
      | [uw vw ww]'
  note: Exclude time-
      | derivatives
      | of windspeeds
  Ftot : Inport
  Mtot : Inport  Port=2
  uwind : Inport  Port=3
  yatm : Inport  Port=4
  yhlp : Inport  Port=5
  " *1" : Gain  SaturateOnIntegerOverflow=on  OutDataTypeStr=Inherit: Same as input  ParamDataTypeStr=Inherit: Same as input
  *1 : Gain  SaturateOnIntegerOverflow=on  OutDataTypeStr=Inherit: Same as input  ParamDataTypeStr=Inherit: Same as input
  Demux : Demux  Outputs=[3 3]
  Discrete-Time Integrator : DiscreteIntegrator  InitialCondition=x0  SampleTime=T  ICPrevOutput=DiscIntNeverNeededParam  ICPrevScaledInput=DiscIntNeverNeededParam
  ODE : Subsystem
  Sum : Sum  SaturateOnIntegerOverflow=on  InputSameDT=on  OutDataTypeStr=Inherit: Same as first input
  Terminator_1 : Terminator
  uvw : Subsystem  mask(uvw){}
      mask help:
      | Calculation of body-axes velocities
      | u, v, and w
      mask Display: disp('Body-axes\nvelocities')
  xdotcorr : Subsystem  mask(xdotcorr){b=GM1(2), S=GM1(3), m=GM1(10), CYbdot=AM(2,19)}
      mask prompts: b "Wing span [m]:"; S "Wing surface [m^2]:"; m "Mass of the aircraft [kg]:"; CYbdot "Stability-derivative CYbdot:"
      mask help:
      | Correction block to write state
      | equations for DHC-2 Beaver aircraft
      | explicitly.
      mask Display: disp('xdotcorr\n(General)')
  xfix : Gain  Gain=xfix  SaturateOnIntegerOverflow=on  OutDataTypeStr=Inherit: Same as input  ParamDataTypeStr=Inherit: Same as input
  x : Outport
  xdot : Outport  Port=2
  ybvel : Outport  Port=3
  wires:
  " *1"/1 -> ODE/1(x)
  xfix/1 -> xdot/1, Discrete-Time Integrator/1
  Discrete-Time Integrator/1 -> *1/1, " *1"/1, x/1
  *1/1 -> uvw/2(x)
  Mtot/1 -> ODE/3(Mtot)
  Ftot/1 -> ODE/2(Ftot)
  yatm/1 -> xdotcorr/3(yatm)
  xdotcorr/1(xdot corrected) -> xfix/1
  Demux/1 -> Sum/1
  uwind/1 -> Demux/1
  uvw/1(ybvel) -> Sum/2, ybvel/1
  Sum/1 -> ODE/5(ybvel*)
  ODE/1(xdot) -> xdotcorr/1(xdot uncorrected)
  yhlp/1 -> xdotcorr/2(yhlp), ODE/4(yhlp), uvw/1(yhlp)
  Demux/2 -> Terminator_1/1

== system model_plane_identification_script_v1/Aircraft Model/Airdata calculation ==
  note: yatm=[rho ps T mu g]
  note: yad1=[soundspeed Mach dynamic_pressure]
  x : Inport
  ad1 : Subsystem  mask(Airdata1){}
      mask help: Basic airdata variables
      mask Display: disp('Airdata1')
  ad2 : Subsystem  mask(Airdata2){}
      mask help: More airdata variables
      mask Display: disp('Airdata2')
  ad3 : Subsystem  mask(Airdata3){cbar=GM1(1)}
      mask prompts: cbar "Mean aerodynamic chord [m]:"
      mask help: More airdata variables
      mask Display: disp('Airdata3')
  atm : Subsystem  mask(Atmosph){}
      mask help: Atmosphere variables
      mask Display: disp('Atmosph')
  yad2 : Terminator
  yad3 : Terminator
  yatm : Outport
  yad1 : Outport  Port=2
  wires:
  ad1/1(yad1) -> ad3/3(yad1), ad2/2(yad1), yad1/1
  atm/1(yatm) -> ad3/2(yatm), ad2/1(yatm), ad1/2(yatm), yatm/1
  x/1 -> ad3/1(x), ad1/1(x), atm/1(x)
  ad3/1(yad3) -> yad3/1
  ad2/1(yad2) -> yad2/1

== system model_plane_identification_script_v1/Aircraft Model/Gravity forces FbMb ==
  x : Inport
  yatm : Inport  Port=2
  Mux : Mux  Inputs=3
  Mux1 : Mux  Inputs=[12 5]
  Xgr : Fcn  Expr=-m*u[17]*sin(u[8])
  Ygr : Fcn  Expr=m*u[17]*cos(u[8])*sin(u[9])
  Zgr : Fcn  Expr=m*u[17]*cos(u[8])*cos(u[9])
  Fgrav : Outport
  wires:
  yatm/1 -> Mux1/2
  x/1 -> Mux1/1
  Zgr/1 -> Mux/3
  Mux1/1 -> Zgr/1, Xgr/1, Ygr/1
  Mux/1 -> Fgrav/1
  Ygr/1 -> Mux/2
  Xgr/1 -> Mux/1

== system model_plane_identification_script_v1/Aircraft Model/Propeller Effects ==
  x : Inport
  Constant : Constant  Value=0
  Mux1 : Mux  Inputs=6
  xt : Terminator
  FMpropeller : Outport
  wires:
  Constant/1 -> Mux1/1, Mux1/2, Mux1/3, Mux1/4, Mux1/5, Mux1/6
  Mux1/1 -> FMpropeller/1
  x/1 -> xt/1

== system model_plane_identification_script_v1/Aircraft Model/Wind forces ==
  x : Inport
  uwind : Inport  Port=2
  -Xw/m : Fcn  Expr=u[16] + u[5]*u[15] - u[6]*u[14]
  -Yw/m : Fcn  Expr=u[17] - u[4]*u[15] + u[6]*u[13]
  -Zw/m : Fcn  Expr=u[18] + u[4]*u[14] - u[5]*u[13]
  Mux : Mux  Inputs=3
  Mux1 : Mux  Inputs=[12 6]
  gain : Gain  Gain=-m  SaturateOnIntegerOverflow=on  OutDataTypeStr=Inherit: Same as input  ParamDataTypeStr=Inherit: Same as input
  Fwind : Outport
  wires:
  -Zw/m/1 -> Mux/3
  -Xw/m/1 -> Mux/1
  -Yw/m/1 -> Mux/2
  Mux1/1 -> -Xw/m/1, -Zw/m/1, -Yw/m/1
  Mux/1 -> gain/1
  gain/1 -> Fwind/1
  x/1 -> Mux1/1
  uwind/1 -> Mux1/2

== system model_plane_identification_script_v1/Aircraft Model/hlpfcn ==
  x : Inport
  Mux : Mux  Inputs=11
  cos alpha : Fcn  Expr=cos(u[2])
  cos beta : Fcn  Expr=cos(u[3])
  cos phi : Fcn  Expr=cos(u[9])
  cos psi : Fcn  Expr=cos(u[7])
  cos theta : Fcn  Expr=cos(u[8])
  sin alpha : Fcn  Expr=sin(u[2])
  sin beta : Fcn  Expr=sin(u[3])
  sin phi : Fcn  Expr=sin(u[9])
  sin psi : Fcn  Expr=sin(u[7])
  sin theta : Fcn  Expr=sin(u[8])
  tan beta : Fcn  Expr=tan(u[3])
  yhlp : Outport
  wires:
  cos phi/1 -> Mux/11
  Mux/1 -> yhlp/1
  sin phi/1 -> Mux/10
  cos theta/1 -> Mux/9
  sin theta/1 -> Mux/8
  cos psi/1 -> Mux/7
  sin psi/1 -> Mux/6
  tan beta/1 -> Mux/5
  sin beta/1 -> Mux/4
  cos beta/1 -> Mux/3
  sin alpha/1 -> Mux/2
  cos alpha/1 -> Mux/1
  x/1 -> cos psi/1, cos phi/1, sin phi/1, cos theta/1, sin theta/1, tan beta/1, cos alpha/1, sin alpha/1, cos beta/1, sin beta/1, sin psi/1

== system model_plane_identification_script_v1/CL/Klg  ==
  In1 : Inport
  Matrix Gain : StateSpace  A=[]  B=[]  C=[]  D=M  X0=0
  Out1 : Outport
  wires:
  In1/1 -> Matrix Gain/1
  Matrix Gain/1 -> Out1/1

== system model_plane_identification_script_v1/CL/Klt  ==
  In1 : Inport
  Matrix Gain : StateSpace  A=[]  B=[]  C=[]  D=M  X0=0
  Out1 : Outport
  wires:
  In1/1 -> Matrix Gain/1
  Matrix Gain/1 -> Out1/1

== system model_plane_identification_script_v1/CL/Manual input ==
  Demux : Demux  Tag=STV Demux  Outputs=1
  FromWs : FromWorkspace  Tag=STV FromWs  VariableName=tuvar  SampleTime=0
      SigBuilderData=|
      | common.afterFinalStr = 'Extrapolate'
      | common.sampleTime = 0
      | dataSet.timeRange = [0 50]
      | dataSet.name = 'Group 1'
      | sbobj.Groups.Name = 'Group 1'
      | sbobj.Groups.Signals.Name = 'deltae_CMD'
      | sbobj.Groups.Signals.XData = [0 15 15 25 25 50]
      | sbobj.Groups.Signals.YData = [0 0 -0.0872664625997 -0.0872664625997 0 0]
      | sbobj.Groups.TimeRange = [0 50]
  deltae_CMD : Outport  Tag=STV Outport
  wires:
  Demux/1 -> deltae_CMD/1
  FromWs/1 -> Demux/1

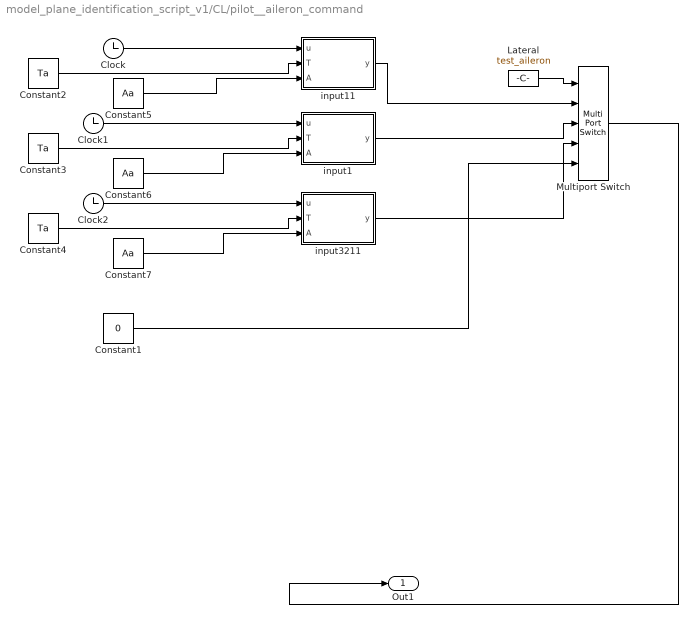
== system model_plane_identification_script_v1/CL/pilot__aileron_command ==
  Clock : Clock
  Clock1 : Clock
  Clock2 : Clock
  Constant1 : Constant  Value=0
  Constant2 : Constant  Value=Ta
  Constant3 : Constant  Value=Ta
  Constant4 : Constant  Value=Ta
  Constant5 : Constant  Value=Aa
  Constant6 : Constant  Value=Aa
  Constant7 : Constant  Value=Aa
  Lateral : Constant  Value=test_aileron
  Multiport Switch : MultiPortSwitch  Inputs=4
  input1 : MATLAB Function  TreatAsAtomicUnit=on
  input11 : MATLAB Function  TreatAsAtomicUnit=on
  input3211 : MATLAB Function  TreatAsAtomicUnit=on
  Out1 : Outport
  wires:
  Constant1/1 -> Multiport Switch/5
  Constant2/1 -> input11/2(T)
  input1/1(y) -> Multiport Switch/3
  Constant4/1 -> input3211/2(T)
  Multiport Switch/1 -> Out1/1
  Lateral/1 -> Multiport Switch/1
  Clock2/1 -> input3211/1(u)
  Constant3/1 -> input1/2(T)
  Clock1/1 -> input1/1(u)
  input11/1(y) -> Multiport Switch/2
  Clock/1 -> input11/1(u)
  input3211/1(y) -> Multiport Switch/4
  Constant5/1 -> input11/3(A)
  Constant6/1 -> input1/3(A)
  Constant7/1 -> input3211/3(A)

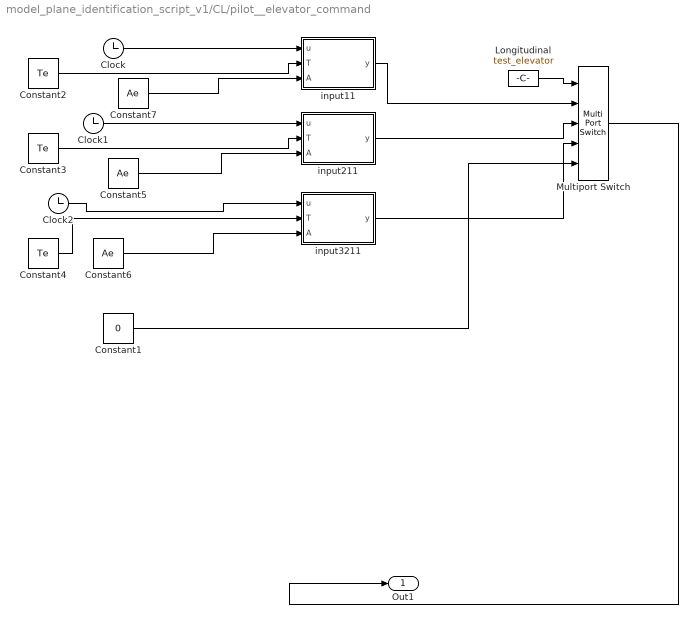
== system model_plane_identification_script_v1/CL/pilot__elevator_command ==
  Clock : Clock
  Clock1 : Clock
  Clock2 : Clock
  Constant1 : Constant  Value=0
  Constant2 : Constant  Value=Te
  Constant3 : Constant  Value=Te
  Constant4 : Constant  Value=Te
  Constant5 : Constant  Value=Ae
  Constant6 : Constant  Value=Ae
  Constant7 : Constant  Value=Ae
  Longitudinal : Constant  Value=test_elevator
  Multiport Switch : MultiPortSwitch  Inputs=4
  input11 : MATLAB Function  TreatAsAtomicUnit=on
  input211 : MATLAB Function  TreatAsAtomicUnit=on
  input3211 : MATLAB Function  TreatAsAtomicUnit=on
  Out1 : Outport
  wires:
  Constant1/1 -> Multiport Switch/5
  Constant2/1 -> input11/2(T)
  input211/1(y) -> Multiport Switch/3
  Constant4/1 -> input3211/2(T)
  Multiport Switch/1 -> Out1/1
  Longitudinal/1 -> Multiport Switch/1
  Clock2/1 -> input3211/1(u)
  Constant3/1 -> input211/2(T)
  Clock1/1 -> input211/1(u)
  input11/1(y) -> Multiport Switch/2
  Clock/1 -> input11/1(u)
  input3211/1(y) -> Multiport Switch/4
  Constant6/1 -> input3211/3(A)
  Constant5/1 -> input211/3(A)
  Constant7/1 -> input11/3(A)

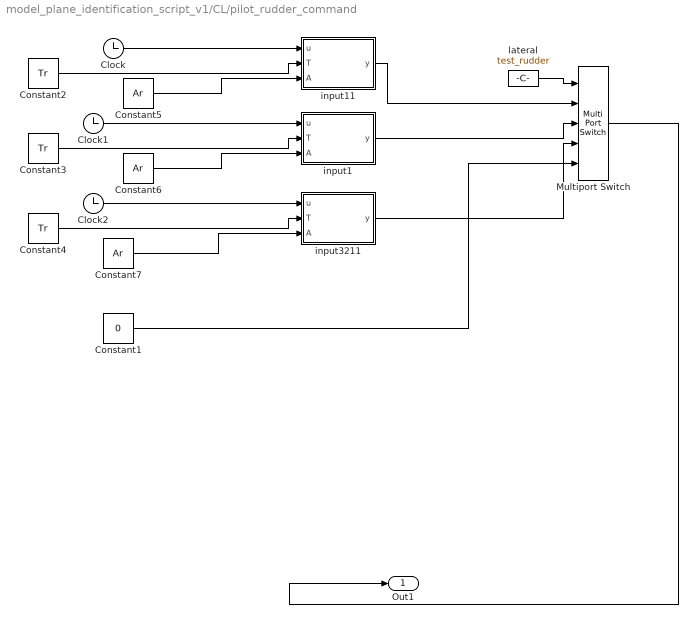
== system model_plane_identification_script_v1/CL/pilot_rudder_command ==
  Clock : Clock
  Clock1 : Clock
  Clock2 : Clock
  Constant1 : Constant  Value=0
  Constant2 : Constant  Value=Tr
  Constant3 : Constant  Value=Tr
  Constant4 : Constant  Value=Tr
  Constant5 : Constant  Value=Ar
  Constant6 : Constant  Value=Ar
  Constant7 : Constant  Value=Ar
  Multiport Switch : MultiPortSwitch  Inputs=4
  input1 : MATLAB Function  TreatAsAtomicUnit=on
  input11 : MATLAB Function  TreatAsAtomicUnit=on
  input3211 : MATLAB Function  TreatAsAtomicUnit=on
  lateral : Constant  Value=test_rudder
  Out1 : Outport
  wires:
  Constant1/1 -> Multiport Switch/5
  Constant2/1 -> input11/2(T)
  input1/1(y) -> Multiport Switch/3
  Constant4/1 -> input3211/2(T)
  Multiport Switch/1 -> Out1/1
  lateral/1 -> Multiport Switch/1
  Clock2/1 -> input3211/1(u)
  Constant3/1 -> input1/2(T)
  Clock1/1 -> input1/1(u)
  input11/1(y) -> Multiport Switch/2
  Clock/1 -> input11/1(u)
  input3211/1(y) -> Multiport Switch/4
  Constant7/1 -> input3211/3(A)
  Constant6/1 -> input1/3(A)
  Constant5/1 -> input11/3(A)

== system model_plane_identification_script_v1/elevator/IIR1 ==
  In : Inport
  Discrete State-Space : DiscreteStateSpace  A=A  B=B  C=C  D=D  X0=x0  SampleTime=T
  Out : Outport
  wires:
  Discrete State-Space/1 -> Out/1
  In/1 -> Discrete State-Space/1

== system model_plane_identification_script_v1/elevator/IIR2 ==
  In : Inport
  Discrete State-Space : DiscreteStateSpace  A=A  B=B  C=C  D=D  X0=x0  SampleTime=T
  Out : Outport
  wires:
  Discrete State-Space/1 -> Out/1
  In/1 -> Discrete State-Space/1

== system model_plane_identification_script_v1/elevator/IIR3 ==
  In : Inport
  Discrete State-Space : DiscreteStateSpace  A=A  B=B  C=C  D=D  X0=x0  SampleTime=T
  Out : Outport
  wires:
  Discrete State-Space/1 -> Out/1
  In/1 -> Discrete State-Space/1

== system model_plane_identification_script_v1/elevator/IIR4 ==
  In : Inport
  Discrete State-Space : DiscreteStateSpace  A=A  B=B  C=C  D=D  X0=x0  SampleTime=T
  Out : Outport
  wires:
  Discrete State-Space/1 -> Out/1
  In/1 -> Discrete State-Space/1

== system model_plane_identification_script_v1/Aircraft Model/Additional outputs/accel ==
  Ftot : Inport
  Fgrav : Inport  Port=2
  Ax : Fcn  Expr=(u[1]-u[4])/(m*9.80665)
  Ay : Fcn  Expr=(u[2]-u[5])/(m*9.80665)
  Az : Fcn  Expr=(u[3]-u[6])/(m*9.80665)
  Mux : Mux  Inputs=6
  Mux1 : Mux  Inputs=[3 3]
  axk : Fcn  Expr=u[1]/(m*9.80665)
  ayk : Fcn  Expr=u[2]/(m*9.80665)
  azk : Fcn  Expr=u[3]/(m*9.80665)
  yacc : Outport
  wires:
  ayk/1 -> Mux/5
  axk/1 -> Mux/4
  Mux1/1 -> ayk/1, azk/1, axk/1, Ay/1, Ax/1, Az/1
  Ax/1 -> Mux/1
  Ay/1 -> Mux/2
  Az/1 -> Mux/3
  azk/1 -> Mux/6
  Mux/1 -> yacc/1
  Fgrav/1 -> Mux1/2
  Ftot/1 -> Mux1/1

== system model_plane_identification_script_v1/Aircraft Model/Additional outputs/fp ==
  x : Inport
  xdot : Inport  Port=2
  Mux : Mux  Inputs=[12 12]
  Mux1 : Mux
  Phi : Fcn  Expr=u[9]*cos(u[8]-alpha0)
  chi : Fcn  Expr=u[3]+u[7]
  fpa : Fcn  Expr=u[13]/9.80665
  gamma : Fcn  Expr=asin(u[24]/u[1])
  yfp : Outport
  wires:
  xdot/1 -> Mux/2
  x/1 -> Mux/1
  Mux1/1 -> yfp/1
  Phi/1 -> Mux1/4
  chi/1 -> Mux1/3
  fpa/1 -> Mux1/2
  Mux/1 -> gamma/1, fpa/1, Phi/1, chi/1
  gamma/1 -> Mux1/1

== system model_plane_identification_script_v1/Aircraft Model/Additional outputs/uvwdot ==
  note: V
  note: sin(beta)
  note: cos(beta)
  note: sin(alpha)
  note: cos(alpha)
  note: `
  x : Inport
  xdot : Inport  Port=2
  yhlp : Inport  Port=3
  DeMux : Demux  Outputs=[1 1 1 1 7]
  Demux : Demux  Outputs=[1 11]
  Mux : Mux  Inputs=[1 1 1 1 1 12]
  Mux1 : Mux  Inputs=3
  Terminator : Terminator
  Terminator1 : Terminator
  u dot : Fcn  Expr=u[6]*u[1]*u[3] - u[5]*(u[7]*u[2]*u[3] + u[8]*u[1]*u[4])
  v dot : Fcn  Expr=u[6]*u[4] + u[5]*u[3]*u[8]
  wdot : Fcn  Expr=u[6]*u[2]*u[3] + u[5]*(u[7]*u[1]*u[3] - u[8]*u[2]*u[4])
  yuvw = [udot; vdot; wdot] : Outport
  wires:
  Demux/1 -> Mux/5
  DeMux/4 -> Mux/4
  DeMux/3 -> Mux/3
  yhlp/1 -> DeMux/1
  Mux1/1 -> yuvw = [udot; vdot; wdot]/1
  x/1 -> Demux/1
  DeMux/2 -> Mux/2
  DeMux/1 -> Mux/1
  Mux/1 -> u dot/1, wdot/1, v dot/1
  xdot/1 -> Mux/6
  u dot/1 -> Mux1/1
  v dot/1 -> Mux1/2
  wdot/1 -> Mux1/3
  DeMux/5 -> Terminator/1
  Demux/2 -> Terminator1/1

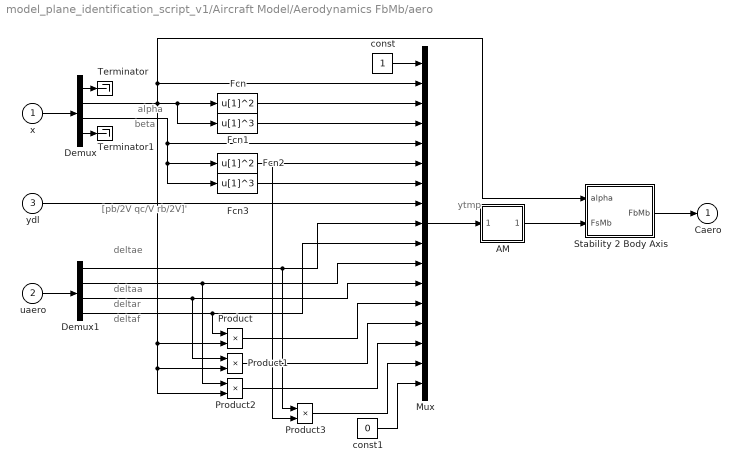
== system model_plane_identification_script_v1/Aircraft Model/Aerodynamics FbMb/aero ==
  note: ytmp
  note: alpha
  note: deltaf
  note: deltar
  note: deltaa
  note: deltae
  note: beta
  note: [pb/2V qc/V rb/2V]'
  x : Inport
  uaero : Inport  Port=2
  ydl : Inport  Port=3
  "AM " : Subsystem  mask(State Space){M=AM}
      mask prompts: M "Matrix"
      mask Display: disp('Matrix\nGain')
  Demux : Demux  Outputs=[1 1 1 9]
  Demux1 : Demux
  Fcn : Fcn  Expr=u[1]^2
  Fcn1 : Fcn  Expr=u[1]^3
  Fcn2 : Fcn  Expr=u[1]^2
  Fcn3 : Fcn  Expr=u[1]^3
  Mux : Mux  Inputs=[1 1 1 1 1 1 1 3 1 1 1 1 1 1 1 1 1]
  Product{,1..3} (4 alike) : Product  SaturateOnIntegerOverflow=on  RndMeth=Zero  InputSameDT=on  OutDataTypeStr=Inherit: Same as first input
  Stability 2 Body Axis : Subsystem
  Terminator : Terminator
  Terminator1 : Terminator
  const : Constant
  const1 : Constant  Value=0
  Caero : Outport
  wires:
  "AM "/1(Out1) -> Stability 2 Body Axis/2(FsMb)
  Stability 2 Body Axis/1(FbMb) -> Caero/1
  Mux/1 -> "AM "/1(In1)
  x/1 -> Demux/1
  Fcn/1 -> Mux/3
  Fcn1/1 -> Mux/4
  uaero/1 -> Demux1/1
  Fcn3/1 -> Mux/7
  Product/1 -> Mux/13
  Demux1/3 -> Product1/1, Mux/12
  Demux1/2 -> Product2/1, Mux/11
  Demux/3 -> Fcn3/1, Fcn2/1, Mux/5
  Demux/2 -> Stability 2 Body Axis/1(alpha), Mux/2, Product2/2, Product1/2, Product/2, Fcn1/1, Fcn/1
  Demux1/4 -> Product/1, Mux/10
  Fcn2/1 -> Product3/2, Mux/6
  Demux1/1 -> Product3/1, Mux/9
  Product1/1 -> Mux/14
  Product2/1 -> Mux/15
  Product3/1 -> Mux/16
  ydl/1 -> Mux/8
  const/1 -> Mux/1
  const1/1 -> Mux/17
  Demux/1 -> Terminator/1
  Demux/4 -> Terminator1/1

== system model_plane_identification_script_v1/Aircraft Model/Aerodynamics FbMb/dl ==
  x : Inport
  Mux : Mux  Inputs=3
  pb/2V : Fcn  Expr=0.5 * u[4] * b / u[1]
  qc/2V : Fcn  Expr=0.5* u[5] * cbar / u[1]
  rb/2V : Fcn  Expr=0.5 * u[6] * b / u[1]
  ydl : Outport
  wires:
  x/1 -> pb/2V/1, rb/2V/1, qc/2V/1
  Mux/1 -> ydl/1
  rb/2V/1 -> Mux/3
  qc/2V/1 -> Mux/2
  pb/2V/1 -> Mux/1
